simulink model "phase2_signal_control_testbench"  (R2025b)
settings: Solver=FixedStepDiscrete  StartTime=0.0  StopTime=80  FixedStep=1  RelTol=1e-3
settings Model: Creator=1234  LastModifiedBy=1234

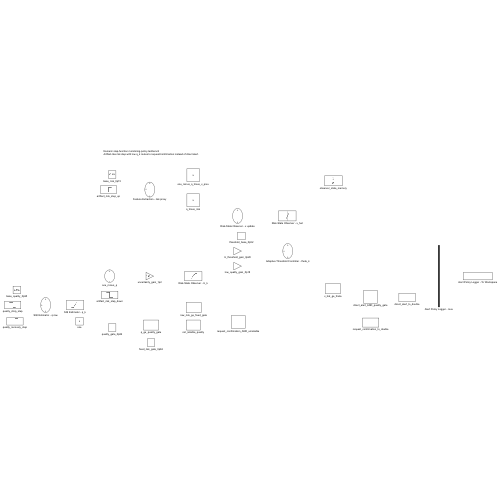
[thumbnail: Simulink's stored preview of the top-level diagram]
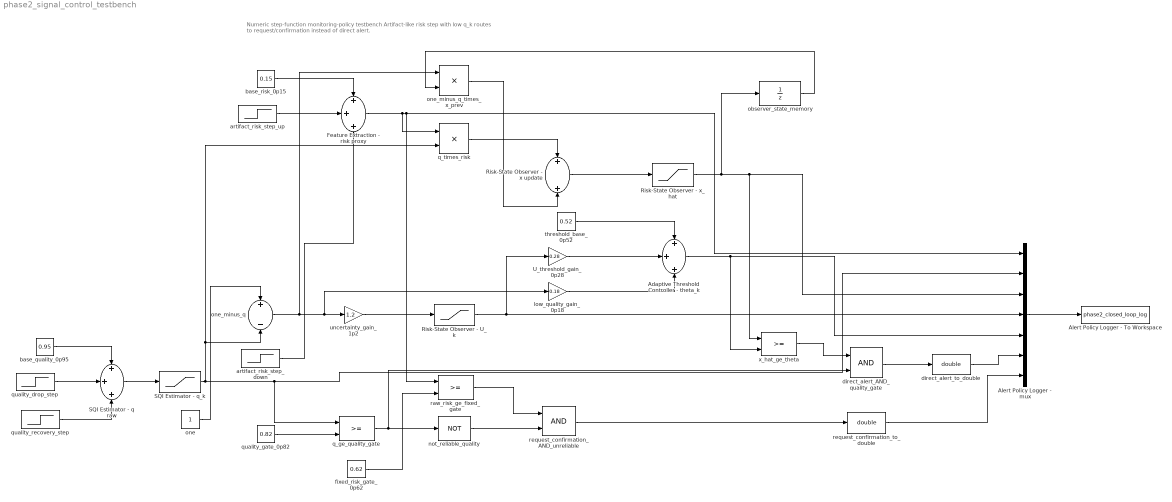
== system phase2_signal_control_testbench ==
  note: Numeric step-function monitoring-policy testbench
      | Artifact-like risk step with low q_k routes to request/confirmation instead of direct alert.
  Adaptive Threshold Controller - theta_k : Sum  Inputs=+++
  Alert Policy Logger - To Workspace : ToWorkspace  VariableName=phase2_closed_loop_log  SaveFormat=Timeseries  SampleTime=-1
  Alert Policy Logger - mux : Mux  Inputs=7
  Feature Extraction - risk proxy : Sum  Inputs=+++
  Risk-State Observer - U_k : Saturate  UpperLimit=1  LowerLimit=0
  Risk-State Observer - x update : Sum
  Risk-State Observer - x_hat : Saturate  UpperLimit=1  LowerLimit=0
  SQI Estimator - q raw : Sum  Inputs=+++
  SQI Estimator - q_k : Saturate  UpperLimit=1  LowerLimit=0
  U_threshold_gain_0p28 : Gain  Gain=0.28
  artifact_risk_step_down : Step  Time=55  After=-0.78  SampleTime=0
  artifact_risk_step_up : Step  Time=20  After=0.78  SampleTime=0
  base_quality_0p95 : Constant  Value=0.95
  base_risk_0p15 : Constant  Value=0.15
  direct_alert_AND_quality_gate : Logic  AllPortsSameDT=off  OutDataTypeStr=boolean
  direct_alert_to_double : DataTypeConversion  OutDataTypeStr=double  SaturateOnIntegerOverflow=off  RndMeth=Floor
  fixed_risk_gate_0p62 : Constant  Value=0.62
  low_quality_gain_0p18 : Gain  Gain=0.18
  not_reliable_quality : Logic  Operator=NOT  AllPortsSameDT=off  OutDataTypeStr=boolean
  observer_state_memory : UnitDelay  InitialCondition=0.15  HasFrameUpgradeWarning=on
  one : Constant
  one_minus_q : Sum  Inputs=+-
  one_minus_q_times_x_prev : Product
  q_ge_quality_gate : RelationalOperator  OutDataTypeStr=boolean  RndMeth=Simplest  InputSameDT=off
  q_times_risk : Product
  quality_drop_step : Step  Time=20  After=-0.42  SampleTime=0
  quality_gate_0p82 : Constant  Value=0.82
  quality_recovery_step : Step  Time=55  After=0.42  SampleTime=0
  raw_risk_ge_fixed_gate : RelationalOperator  OutDataTypeStr=boolean  RndMeth=Simplest  InputSameDT=off
  request_confirmation_AND_unreliable : Logic  AllPortsSameDT=off  OutDataTypeStr=boolean
  request_confirmation_to_double : DataTypeConversion  OutDataTypeStr=double  SaturateOnIntegerOverflow=off  RndMeth=Floor
  threshold_base_0p52 : Constant  Value=0.52
  uncertainty_gain_1p2 : Gain  Gain=1.2
  x_hat_ge_theta : RelationalOperator  OutDataTypeStr=boolean  RndMeth=Simplest  InputSameDT=off
  wires:
  base_quality_0p95/1 -> SQI Estimator - q raw/1
  quality_recovery_step/1 -> SQI Estimator - q raw/3
  SQI Estimator - q raw/1 -> SQI Estimator - q_k/1
  quality_drop_step/1 -> SQI Estimator - q raw/2
  one_minus_q/1 -> low_quality_gain_0p18/1, uncertainty_gain_1p2/1, one_minus_q_times_x_prev/1
  one/1 -> one_minus_q/1
  SQI Estimator - q_k/1 -> q_ge_quality_gate/1, Alert Policy Logger - mux/2, q_times_risk/2, one_minus_q/2
  base_risk_0p15/1 -> Feature Extraction - risk proxy/1
  artifact_risk_step_up/1 -> Feature Extraction - risk proxy/2
  artifact_risk_step_down/1 -> Feature Extraction - risk proxy/3
  q_ge_quality_gate/1 -> direct_alert_AND_quality_gate/2, not_reliable_quality/1
  quality_gate_0p82/1 -> q_ge_quality_gate/2
  Feature Extraction - risk proxy/1 -> Alert Policy Logger - mux/1, raw_risk_ge_fixed_gate/1, q_times_risk/1
  uncertainty_gain_1p2/1 -> Risk-State Observer - U_k/1
  not_reliable_quality/1 -> request_confirmation_AND_unreliable/2
  raw_risk_ge_fixed_gate/1 -> request_confirmation_AND_unreliable/1
  fixed_risk_gate_0p62/1 -> raw_risk_ge_fixed_gate/2
  Risk-State Observer - x update/1 -> Risk-State Observer - x_hat/1
  q_times_risk/1 -> Risk-State Observer - x update/1
  one_minus_q_times_x_prev/1 -> Risk-State Observer - x update/2
  Adaptive Threshold Controller - theta_k/1 -> Alert Policy Logger - mux/5, x_hat_ge_theta/2
  low_quality_gain_0p18/1 -> Adaptive Threshold Controller - theta_k/3
  Risk-State Observer - U_k/1 -> Alert Policy Logger - mux/4, U_threshold_gain_0p28/1
  threshold_base_0p52/1 -> Adaptive Threshold Controller - theta_k/1
  U_threshold_gain_0p28/1 -> Adaptive Threshold Controller - theta_k/2
  request_confirmation_AND_unreliable/1 -> request_confirmation_to_double/1
  Risk-State Observer - x_hat/1 -> Alert Policy Logger - mux/3, x_hat_ge_theta/1, observer_state_memory/1
  observer_state_memory/1 -> one_minus_q_times_x_prev/2
  x_hat_ge_theta/1 -> direct_alert_AND_quality_gate/1
  direct_alert_AND_quality_gate/1 -> direct_alert_to_double/1
  request_confirmation_to_double/1 -> Alert Policy Logger - mux/7
  direct_alert_to_double/1 -> Alert Policy Logger - mux/6
  Alert Policy Logger - mux/1 -> Alert Policy Logger - To Workspace/1
